simulink model "testPlatform"  (R2018b)
settings: Solver=VariableStepAuto  StartTime=0.0  StopTime=simTime/2  RelTol=1e-3
values from neighbouring files (symbols this model uses):
  basisVec = linspace(0,20,size_grid)*(pi/180)    [rgpTestAyaz.m]    (also in rgpTestWind.m = heights(:)'; testRgpKf.m = [heights(:)'; zeros(1,numel(heights))])
  hMax = 1500    [rgpTestWind.m]    (also in testGPKF.m; testGenWind.m; testRgpKf.m; testSEGPKF.m)
  hMin = 100    [rgpTestWind.m]    (also in testGPKF.m; testGenWind.m; testRgpKf.m; testSEGPKF.m)
  hyperParams = optHyperParams    [rgpTestWind.m]    (also in testGPKF.m = [hyp.funcVar;hyp.lengthScale;hyp.timeScale;hyp.noiseVariance; testRgpKf.m = [hyp.funcVar;hyp.noiseVariance;hyp.lengthScale;hyp.timeScale; testSEGPKF.m = [1 heightScale timeScale 0*0.0001]')
  initInvCovMat = inv(initCovMat + (1e-5)*eye(size_grid))    [rgpTestAyaz.m]    (also in rgpTestWind.m = inv(initCovMat + optHyperParams(2)*eye(noTP)))
undefined symbols (not defined in the file or in its folder): initCovMat, initMeanVec
libraries: dspmtrx3 x1, simulink x1
settings Model: Creator=Ayaz  LastModifiedBy=Ayaz

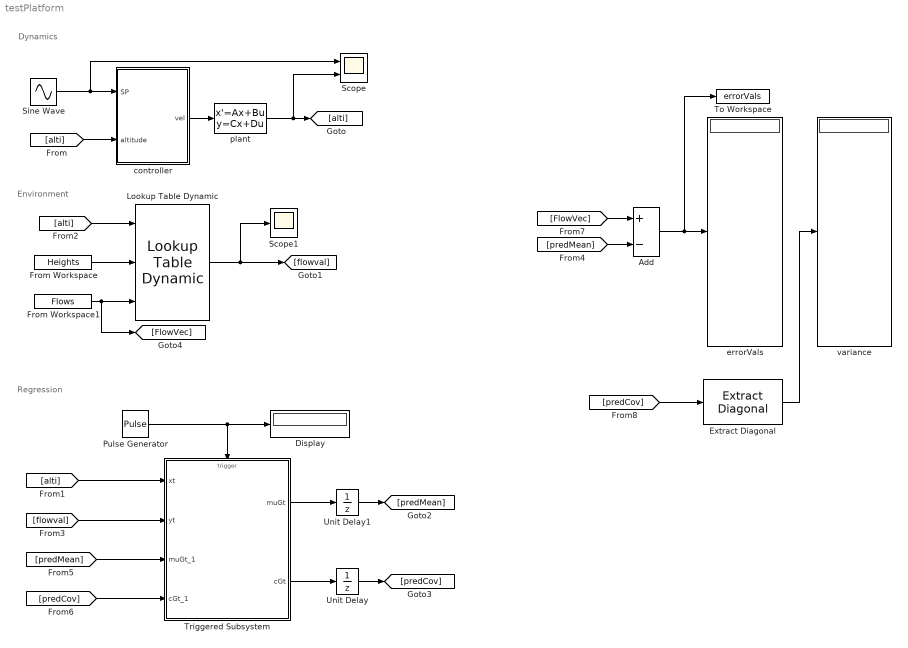
== system testPlatform ==
  note: Dynamics
  note: Environment
  note: Regression
  Add : Sum  Inputs=+-
  Display : Display
  Extract Diagonal : dspmtrx3/Extract Diagonal
      settings: SourceProductName=DSP System Toolbox  SourceProductBaseCode=DS
  From Workspace : FromWorkspace  VariableName=Heights  SampleTime=0
  From Workspace1 : FromWorkspace  VariableName=Flows  SampleTime=0
  Lookup Table Dynamic : simulink/Lookup Tables/Lookup Table Dynamic  LookUpMeth=Interpolation-Use End Values  OutDataType=fixdt('double')  OutScaling=[]  OutputDataTypeScalingMode=Specify via dialog  OutDataTypeStr=double  DoSatur=off
      settings: SourceProductName=Simulink
  Pulse Generator : DiscretePulseGenerator  PulseType=Time based  Period=1  PulseWidth=50
  Scope : Scope  NumInputPorts=2
  Scope1 : Scope
  Sine Wave : Sin  Amplitude=0.5*(hMax-hMin)  Bias=0.5*(hMax-hMin)  Frequency=2*pi*0.01  SampleTime=0
  To Workspace : ToWorkspace  VariableName=errorVals  SaveFormat=Timeseries  SampleTime=-1
  Triggered Subsystem : Subsystem  TreatAsAtomicUnit=on
  Unit Delay : UnitDelay  InitialCondition=initCovMat  SampleTime=-1
  Unit Delay1 : UnitDelay  InitialCondition=initMeanVec  SampleTime=-1
  controller : Subsystem
  errorVals : Display
  plant : StateSpace  A=0  D=0  InitialCondition=100
  variance : Display
  wires:
  controller/1(vel) -> plant/1
  plant/1 -> Scope/2, [alti]
  [alti] -> controller/2(altitude)
  Sine Wave/1 -> Scope/1, controller/1(SP)
  [alti] -> Triggered Subsystem/1(xt)
  [alti] -> Lookup Table Dynamic/1
  From Workspace/1 -> Lookup Table Dynamic/2
  From Workspace1/1 -> [FlowVec], Lookup Table Dynamic/3
  Lookup Table Dynamic/1 -> [flowval], Scope1/1
  [flowval] -> Triggered Subsystem/2(yt)
  [predMean] -> Add/2
  Add/1 -> errorVals/1, To Workspace/1
  [predCov] -> Triggered Subsystem/4(cGt_1)
  [predMean] -> Triggered Subsystem/3(muGt_1)
  Triggered Subsystem/1(muGt) -> Unit Delay1/1
  Unit Delay1/1 -> [predMean]
  Triggered Subsystem/2(cGt) -> Unit Delay/1
  Unit Delay/1 -> [predCov]
  [FlowVec] -> Add/1
  [predCov] -> Extract Diagonal/1
  Extract Diagonal/1 -> variance/1
  Pulse Generator/1 -> Display/1, Triggered Subsystem/Trigger

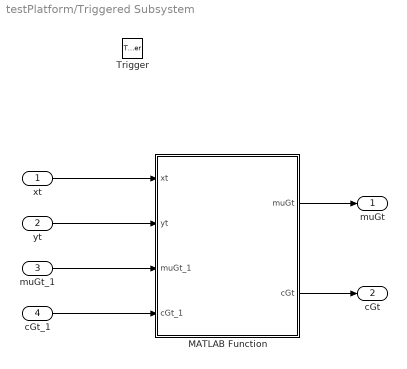
== system testPlatform/Triggered Subsystem ==
  xt : Inport
  yt : Inport  Port=2
  muGt_1 : Inport  Port=3
  cGt_1 : Inport  Port=4
  Trigger : TriggerPort  VariantControl=Variant
  MATLAB Function : MATLAB Function  TreatAsAtomicUnit=on
  muGt : Outport
  cGt : Outport  Port=2
  wires:
  cGt_1/1 -> MATLAB Function/4(cGt_1)
  muGt_1/1 -> MATLAB Function/3(muGt_1)
  yt/1 -> MATLAB Function/2(yt)
  xt/1 -> MATLAB Function/1(xt)
  MATLAB Function/1(muGt) -> muGt/1
  MATLAB Function/2(cGt) -> cGt/1

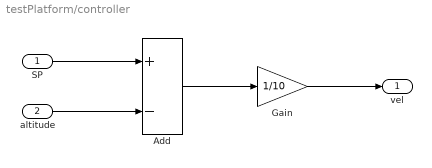
== system testPlatform/controller ==
  SP : Inport
  altitude : Inport  Port=2
  Add : Sum  Inputs=+-
  Gain : Gain  Gain=1/10
  vel : Outport
  wires:
  SP/1 -> Add/1
  altitude/1 -> Add/2
  Add/1 -> Gain/1
  Gain/1 -> vel/1

== matlab function testPlatform/Triggered Subsystem/MATLAB Function ==
  data: xt input; muGt output; yt input; cGt output; hyperParams parameter; basisVec parameter; initMeanVec parameter; initInvCovMat parameter; muGt_1 input; cGt_1 input
function [muGt,cGt] = rgpRegression(xt,yt,hyperParams,...
    basisVec,initMeanVec,initInvCovMat,muGt_1,cGt_1)
% extract values from initialization structure
x = basisVec;
mX = initMeanVec;
invkXX = initInvCovMat;
% number of design/training points
noTP = size(x,2);
% calculate mean and covariance at candidate point
mXt = calcMean(xt);
kXtXt = calcCovariance(xt,xt,hyperParams);
% calculate covariance of candidate wrt design points
kXtX = NaN(1,noTP);
for ii = 1:noTP
    kXtX(1,ii) = calcCovariance(xt,x(:,ii),hyperParams);
end
% calculate Jt as per Huber Eqn. (8)
Jt = kXtX*invkXX;
% calculate B as per Huber Eqn. (7)
B = kXtXt - Jt*kXtX';
% calculate muP as per Huber Eqn. (6)
muP = mXt + Jt*(muGt_1 - mX);
% calculate cP as per Huber Eqn. (9)
cP = B + Jt*cGt_1*Jt';
% calculate Gt (kalman gain matrix) as per Huber Eqn. (12)
Gt = cGt_1*Jt'*(cP + hyperParams(2))^-1;
% calculate mean at step t as per Huber Eqn. (10)
muGt = muGt_1 + Gt*(yt - muP);
% calculate covariance at step t as per Huber Eqn. (11)
cGt = cGt_1 - Gt*Jt*cGt_1;

end

function val = calcCovariance(x1,x2,hyperParams)
% variance of latent function
alphaSquared = hyperParams(1);
% length scales
lengthScales = hyperParams(3:size(x1,1)+2);
% calculate covariance
val = alphaSquared*exp(-0.5*(x1-x2)'*...
    (eye(length(lengthScales))./lengthScales.^2)*(x1-x2));
end

function val = calcMean(x)
% calculate mean
val = 0*(x'*x);
end
